simulink subsystem "AutomaticTransmissionWithTorqueConverterSSC"  (R2023b)
settings: Solver=VariableStepAuto  StartTime=0.0  StopTime=10.0  RelTol=1e-3
undefined symbols (not defined in the file): PlntTransDampVect, PlntTransEffVect, PlntTransGearNumVect, PlntTransGearRatioVect, PlntTrqConvrtrImpDamp, PlntTrqConvrtrTurbDamp
libraries: fl_lib x11, sdl_lib x5, nesl_utility x4, nesl_utility_internal x3, autolibpowerinfoutils x1, autolibsharedcommon x1
settings Model: Creator=The MathWorks, Inc.  LastModifiedBy=The MathWorks, Inc.
settings OptimizationCC: ReuseModelBlockBuffer=off
settings DebuggingCC: SubsystemReferenceDiagnosticForUnitTest=warning

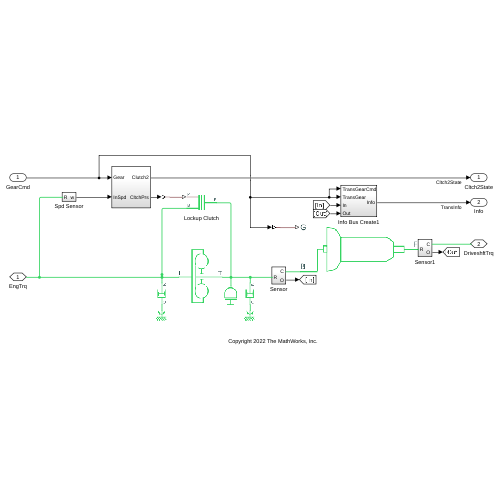
[thumbnail: Simulink's stored preview of the top-level diagram]
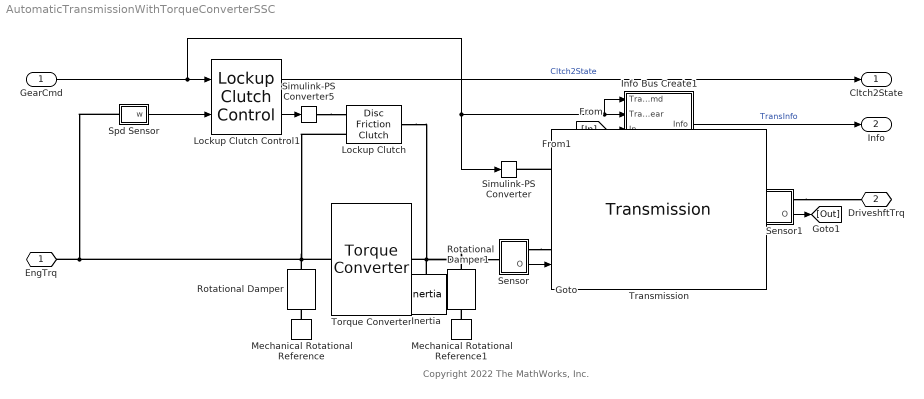
== system AutomaticTransmissionWithTorqueConverterSSC ==
  note: Copyright 2022 The MathWorks, Inc.
  GearCmd : Inport
  Inertia : fl_lib/Mechanical/Rotational Elements/Inertia  inertia=PlntTrqConvrtrTurbInertia kg*m^2  num_ports=foundation.enum.numPorts2.one  w_specify=off  w_priority=High  w=0 rad/s  w_nominal_specify=off  w_nominal_unit=rad/s  w_nominal_value=1  t_specify=off  t_priority=None  t=0 N*m  t_nominal_specify=off  t_nominal_unit=N*m  t_nominal_value=1
  Info Bus Create1 : Subsystem
  Lockup Clutch : sdl_lib/Clutches/Disc Friction Clutch  geometry_model=sdl.enum.friction_geometry.radius  r_eff=PlntTrqConvrtrCltchRadius m  d_o=150 mm  d_i=100 mm  nS=PlntTrqConvrtrCltchNumFricSurf  piston_area=PlntTrqConvrtrCltchEngdPstnArea m^2  unidirectional=sdl.enum.directionality.bidirectional  friction_model=sdl.enum.friction_model_TLU_thermal.fixed  mu_w_vector=[0, 100, 1000] rad/s  temperature_TLU=[280, 300, 320] K  mu_static=PlntTrqConvrtrCltchStatFric  mu_static_vector=[.4, .38, .36]  mu_coulomb=PlntTrqConvrtrCltchKinFric  mu_coulomb_vector=[.3, .22, .19]  mu_coulomb_temp_vector=[.3, .28, .25]  mu_coulomb_matrix=[.34, .32, .3; .3, .28, .25; .25, .2, .15]  mu_interp_method=simscape.enum.interpolation.linear  mu_extrap_method=simscape.enum.extrapolation.linear  d_f=PlntTrqConvrtrCltchDerateFctr  w_tol=PlntTrqConvrtrCltchVelTol rad/s  pressure_min=PlntTrqConvrtrCltchEngdThreshPrs Pa  mu_visc=PlntTrqConvrtrCltchViscDragTrq N*m/(rad/s)  initial_state_locked=sdl.enum.initial_lock.unlocked  enable_faults=simscape.enum.onoff.off  fault_type=sdl.enum.clutchFault.lock  external_fault=simscape.enum.onoff.off  temporal_fault=simscape.enum.onoff.off  fault_time=5 s  report_fault=simscape.enum.assert.action.none  thermal_mass=25 kJ/K  T_init=300 K
      settings: InternalSimscapePortConfiguration="{\"Bottom\":[],\"Left\":[{\"id\":\"P\",\"label\":\"P\",\"type\":\"input\"},{\"id\":\"B\",\"label\":\"B\",\"type\":\"foundation.mechanical.rotational.rotational\"}],\"Right\":[{\"id\":\"F\",\"label\":\"F\",\"type\":\"foundation.mechanical.rotational.rotational\"}],\"Top\":[]}"
  Lockup Clutch Control1 : autolibsharedcommon/Lockup Clutch Control  SystemSampleTime=-1  VariantActivationTime=update diagram  AllowFlexibleInterface=on  Latency=0  AutoFrameSizeCalculation=off
  Mechanical Rotational Reference : fl_lib/Mechanical/Rotational Elements/Mechanical Rotational Reference
  Mechanical Rotational Reference1 : fl_lib/Mechanical/Rotational Elements/Mechanical Rotational Reference
  Rotational Damper : sdl_lib/Couplings & Drives/Springs & Dampers/Rotational Damper  D=PlntTrqConvrtrImpDamp N*m*s/rad  enable_faults=simscape.enum.onoff.off  b_fault=100 N*m*s/rad  temporal_fault=simscape.enum.onoff.off  fault_time=5 s  shock_fault=simscape.enum.onoff.off  acceleration_limit=100 rad/s^2  shock_limit=1  report_fault=simscape.enum.assert.action.none  thermal_port=simscape.enum.thermaleffects.omit  thermal_mass=50 kJ/K  temperature_specify=off  temperature_priority=High  temperature=300 K  temperature_nominal_specify=off  temperature_nominal_unit=K  temperature_nominal_value=1
  Rotational Damper1 : sdl_lib/Couplings & Drives/Springs & Dampers/Rotational Damper  D=PlntTrqConvrtrTurbDamp N*m*s/rad  enable_faults=simscape.enum.onoff.off  b_fault=100 N*m*s/rad  temporal_fault=simscape.enum.onoff.off  fault_time=5 s  shock_fault=simscape.enum.onoff.off  acceleration_limit=100 rad/s^2  shock_limit=1  report_fault=simscape.enum.assert.action.none  thermal_port=simscape.enum.thermaleffects.omit  thermal_mass=50 kJ/K  temperature_specify=off  temperature_priority=High  temperature=300 K  temperature_nominal_specify=off  temperature_nominal_unit=K  temperature_nominal_value=1
  Sensor : Subsystem
      settings: PortSchema="{\"entries\":[{\"content\":{\"sides\":[{\"content\":{\"connectorIds\":[\"LConn1\"]},\"type\":\"ConnectorPlacement.EquallySpacedRectSide\",\"uuid\":\"2e27b447-89d7-4d94-b9d2-8f612a4e25ed\"},{\"content\":{\"connectorIds\":[\"RConn1\",\"Out1\"],\"side\":\"RIGHT\"},\"type\":\"ConnectorPlacement.EquallySpacedRectSide\",\"uuid\":\"d649ff29-a00c-460e-9e09-fe3bc3dd9339\"},{\"content\":{\"side\":\"TOP\"},\"type\":\"ConnectorPlacement.EquallySpacedRectSide\",\"uuid\":\"c1caa1bf-44c8-4179-bd35-f8aecae525f1\"}]},\"type\":\"ConnectorPlacement.EquallySpacedConnector\",\"uuid\":\"741ea5ec-6556-46e5-ba1b-80e523f861d6\"}],\"packageUris\":[\"http://schema.mathworks.com/mf0/Connector/R2020b\"],\"version\":\"1.0\"}"
  Sensor1 : Subsystem
      settings: PortSchema="{\"entries\":[{\"content\":{\"sides\":[{\"content\":{\"connectorIds\":[\"LConn1\"]},\"type\":\"ConnectorPlacement.EquallySpacedRectSide\",\"uuid\":\"2e27b447-89d7-4d94-b9d2-8f612a4e25ed\"},{\"content\":{\"connectorIds\":[\"RConn1\",\"Out1\"],\"side\":\"RIGHT\"},\"type\":\"ConnectorPlacement.EquallySpacedRectSide\",\"uuid\":\"d649ff29-a00c-460e-9e09-fe3bc3dd9339\"},{\"content\":{\"side\":\"TOP\"},\"type\":\"ConnectorPlacement.EquallySpacedRectSide\",\"uuid\":\"c1caa1bf-44c8-4179-bd35-f8aecae525f1\"}]},\"type\":\"ConnectorPlacement.EquallySpacedConnector\",\"uuid\":\"741ea5ec-6556-46e5-ba1b-80e523f861d6\"}],\"packageUris\":[\"http://schema.mathworks.com/mf0/Connector/R2020b\"],\"version\":\"1.0\"}"
  Simulink-PS Converter : nesl_utility_internal/Simulink-PS Converter  PhysicalDomain=network_engine_domain  SubClassName=ps_input  LeftPortType=input  RightPortType=output  PseudoPeriodic=off  Frequencies=[]  NoiseDistribution=none  NoiseParameters=[]  Unit=1  AffineConversion=off  FilteringAndDerivatives=provide  SimscapeFilterOrder=1  InputFilterTimeConstant=0.001  UdotUserProvided=0
  Simulink-PS Converter5 : nesl_utility_internal/Simulink-PS Converter  PhysicalDomain=network_engine_domain  SubClassName=ps_input  LeftPortType=input  RightPortType=output  PseudoPeriodic=off  Frequencies=[]  NoiseDistribution=none  NoiseParameters=[]  Unit=Pa  AffineConversion=off  FilteringAndDerivatives=provide  SimscapeFilterOrder=1  InputFilterTimeConstant=0.01  UdotUserProvided=0
  Spd Sensor : Subsystem
  Torque Converter : sdl_lib/Couplings & Drives/Torque Converter  coast_mode_modeling=sdl.enum.torqueConverterContinuousTwomode.continuous  SR_drive_tlu=PlntTrqConvrtrDrvModeSpdRatioVect  TR_drive_tlu=PlntTrqConvrtrDrvModeTrqRatioVect  CF_drive_tlu=PlntTrqConvrtrDrvModeCapFctrVect N*m/rpm^2  SR_coast_tlu=PlntTrqConvrtrCoastModeSpdRatioVect  CF_coast_tlu=PlntTrqConvrtrCoastModeCapFctrRatioVect N*m/rpm^2  iniMode=sdl.enum.torqueConverterInitialMode.drive  delta_w=PlntTrqConvrtrModeTransThresh rpm  n_vector=PlntTrqConvrtrSpdRatioVect  trq_vector=PlntTrqConvrtrTrqRatioVect  cf_vector_parameterization=sdl.enum.torqueConverterCFParameterization.SpeedToSqrtTorque  cf_vector_reference_speed=sdl.enum.torqueConverterCFReferenceSpeed.ImpellerSpeedAlways  cf_vector=PlntTrqConvrtrCapVect rad/(N^(1/2)*m^(1/2)*s)  cf_vector_sq=1e-3 * [6.616, 6.048, 5.787, 5.384, 4.681, 3.779, 2.671, 2.047, 1.111, .4] N*m*s^2/rad^2  interp_method=simscape.enum.interpolation.smooth  extrap_method=simscape.enum.extrapolation.nearest  model_lag=sdl.enum.torqueConverterLagOnOff.LagOff  tau=PlntTrqConvrtrTimeCnst s  initial_trq_ratio=PlntTrqConvrtrInitTrqRatio
      settings: InternalSimscapePortConfiguration="{\"Bottom\":[],\"Left\":[{\"id\":\"I\",\"label\":\"I\",\"type\":\"foundation.mechanical.rotational.rotational\"}],\"Right\":[{\"id\":\"T\",\"label\":\"T\",\"type\":\"foundation.mechanical.rotational.rotational\"}],\"Top\":[]}"
  Transmission : sdl_lib/Gears/Transmission  gear_ratios=PlntTransGearRatioVect(2:end)  reverse_ratio=PlntTransRvrseGearRatio  friction_model=sdl.enum.transmissionFriction.gear  efficiency=0.95  efficiency_tlu=PlntTransEffVect(2:end)  reverse_efficiency=PlntTransRvrseGearEff  pwr_thr=PlntTransPwrThresh W  kp=PlntTransStiff N*m/rad  kv=PlntTransDamp N*m*s/rad  initial_torque=PlntTransInitInTrq N*m  mu_visc=[PlntTransDampVect(1), PlntTransDampVect(1)] N*m*s/rad  t_friction=PlntTransCltchKinFricTrq N*m  t_locked=PlntTransCltchStatFricTrq N*m  shift_model=sdl.enum.transmissionShiftModel.instant  shift_time=PlntTransCltchShiftTime ms  w_tol=PlntTransCltchVelTol rad/s  initial_state_locked=sdl.enum.initial_lock.locked  thermal_port=simscape.enum.thermaleffects.omit  thermal_mass=100 kJ/K  initial_temperature=300 K
      settings: LogSimulationData=on  InternalSimscapePortConfiguration="{\"Bottom\":[],\"Left\":[{\"id\":\"G\",\"label\":\"G\",\"type\":\"input\"},{\"id\":\"B\",\"label\":\"B\",\"type\":\"foundation.mechanical.rotational.rotational\"}],\"Right\":[{\"id\":\"F\",\"label\":\"F\",\"type\":\"foundation.mechanical.rotational.rotational\"}],\"Top\":[]}"
  EngTrq : PMIOPort  Side=Left
  DriveshftTrq : PMIOPort  Port=2  Side=Right
  Cltch2State : Outport  VectorParamsAs1DForOutWhenUnconnected=off
  Info : Outport  Port=2  VectorParamsAs1DForOutWhenUnconnected=off
  wires:
  Info Bus Create1/1(Info) -> Info/1  "TransInfo"
  Lockup Clutch Control1/1 -> Cltch2State/1  "Cltch2State"
  GearCmd/1 -> Lockup Clutch Control1/1, Info Bus Create1/1(TransGearCmd), Info Bus Create1/2(TransGear), Simulink-PS Converter/1
  Lockup Clutch Control1/2 -> Simulink-PS Converter5/1
  Spd Sensor/1(w) -> Lockup Clutch Control1/2
  Sensor/1(O) -> [In]
  Sensor1/1(O) -> [Out]
  [In] -> Info Bus Create1/3(In)
  [Out] -> Info Bus Create1/4(Out)
  connections:
  Torque Converter/LConn1 -- Spd Sensor/LConn1 -- EngTrq/RConn1 -- Rotational Damper/LConn1 -- Lockup Clutch/LConn2
  Transmission/LConn1 -- Simulink-PS Converter/RConn1
  Mechanical Rotational Reference/LConn1 -- Rotational Damper/RConn1
  Mechanical Rotational Reference1/LConn1 -- Rotational Damper1/RConn1
  Simulink-PS Converter5/RConn1 -- Lockup Clutch/LConn1
  Lockup Clutch/RConn1 -- Rotational Damper1/LConn1 -- Sensor/LConn1 -- Torque Converter/RConn1 -- Inertia/LConn1
  Sensor1/LConn1 -- Transmission/RConn1
  Sensor/RConn1 -- Transmission/LConn2
  Sensor1/RConn1 -- DriveshftTrq/RConn1

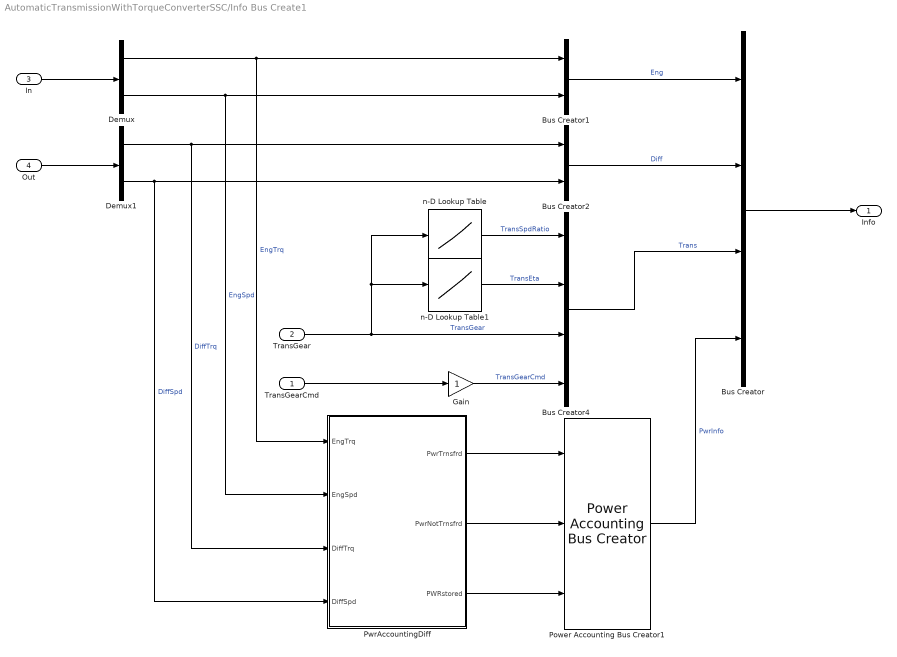
== system AutomaticTransmissionWithTorqueConverterSSC/Info Bus Create1 ==
  TransGearCmd : Inport
  TransGear : Inport  Port=2
  In : Inport  Port=3
  Out : Inport  Port=4
  Bus Creator : BusCreator  Inputs=4
  Bus Creator1 : BusCreator  Inputs=2
  Bus Creator2 : BusCreator  Inputs=2
  Bus Creator4 : BusCreator  Inputs=4
  Demux : Demux  Outputs=2
  Demux1 : Demux  Outputs=2
  Gain : Gain
  Power Accounting Bus Creator1 : autolibpowerinfoutils/Power Accounting Bus Creator  AssctBlkSelPopup=Parent  RefBlkName='libraryname/blkname'  PwrTrnsfrdCheckBox=on  PwrNotTrnsfrdCheckBox=on  PwrStoredCheckBox=on  aMode=aMode
  PwrAccountingDiff : Subsystem
  n-D Lookup Table : Lookup_n-D  NumberOfTableDimensions=1  BreakpointsForDimension1=PlntTransGearNumVect  BreakpointsForDimension3=[5, 7]  BeginIndexSearchUsingPreviousIndexResult=on  Table=PlntTransGearRatioVect  InterpMethod=Nearest  ExtrapMethod=Clip  UseLastTableValue=on  InternalRulePriority=Speed  RndMeth=Simplest
  n-D Lookup Table1 : Lookup_n-D  NumberOfTableDimensions=1  BreakpointsForDimension1=PlntTransGearNumVect  BreakpointsForDimension3=[5, 7]  BeginIndexSearchUsingPreviousIndexResult=on  Table=PlntTransEffVect  InterpMethod=Nearest  ExtrapMethod=Clip  UseLastTableValue=on  InternalRulePriority=Speed  RndMeth=Simplest
  Info : Outport
  wires:
  TransGearCmd/1 -> Gain/1
  PwrAccountingDiff/1(PwrTrnsfrd) -> Power Accounting Bus Creator1/1
  PwrAccountingDiff/3(PWRstored) -> Power Accounting Bus Creator1/3
  PwrAccountingDiff/2(PwrNotTrnsfrd) -> Power Accounting Bus Creator1/2
  Out/1 -> Demux1/1
  In/1 -> Demux/1
  Bus Creator4/1 -> Bus Creator/3  "Trans"
  Power Accounting Bus Creator1/1 -> Bus Creator/4  "PwrInfo"
  Demux1/2 -> Bus Creator2/2, PwrAccountingDiff/4(DiffSpd)  "DiffSpd"
  n-D Lookup Table1/1 -> Bus Creator4/2  "TransEta"
  Bus Creator1/1 -> Bus Creator/1  "Eng"
  Demux/2 -> Bus Creator1/2, PwrAccountingDiff/2(EngSpd)  "EngSpd"
  Demux1/1 -> Bus Creator2/1, PwrAccountingDiff/3(DiffTrq)  "DiffTrq"
  Bus Creator/1 -> Info/1
  n-D Lookup Table/1 -> Bus Creator4/1  "TransSpdRatio"
  Demux/1 -> Bus Creator1/1, PwrAccountingDiff/1(EngTrq)  "EngTrq"
  TransGear/1 -> n-D Lookup Table/1, n-D Lookup Table1/1, Bus Creator4/3  "TransGear"
  Bus Creator2/1 -> Bus Creator/2  "Diff"
  Gain/1 -> Bus Creator4/4  "TransGearCmd"

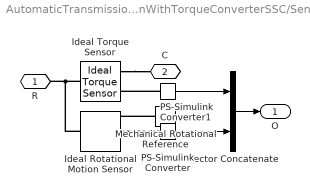
== system AutomaticTransmissionWithTorqueConverterSSC/Sensor ==
  Ideal Rotational Motion Sensor : fl_lib/Mechanical/Mechanical Sensors/Ideal Rotational Motion Sensor  reference=foundation.enum.MeasurementReference.difference  acceleration_port=false  velocity_port=true  position_port=true  wrap_angle=false  offset=0 rad
  Ideal Torque Sensor : fl_lib/Mechanical/Mechanical Sensors/Ideal Torque Sensor
  Mechanical Rotational Reference : fl_lib/Mechanical/Rotational Elements/Mechanical Rotational Reference
  PS-Simulink Converter : nesl_utility/PS-Simulink Converter  PhysicalDomain=network_engine_domain  SubClassName=ps_output  LeftPortType=input  RightPortType=output  PseudoPeriodic=off  Frequencies=[]  VectorFormat=inherit  Unit=inherit  AffineConversion=off
  PS-Simulink Converter1 : nesl_utility/PS-Simulink Converter  PhysicalDomain=network_engine_domain  SubClassName=ps_output  LeftPortType=input  RightPortType=output  PseudoPeriodic=off  Frequencies=[]  VectorFormat=inherit  Unit=inherit  AffineConversion=off
  Vector Concatenate : Concatenate
  R : PMIOPort  Side=Left
  C : PMIOPort  Port=2  Side=Right
  O : Outport
  wires:
  PS-Simulink Converter1/1 -> Vector Concatenate/1
  PS-Simulink Converter/1 -> Vector Concatenate/2
  Vector Concatenate/1 -> O/1
  connections:
  PS-Simulink Converter1/LConn1 -- Ideal Torque Sensor/RConn2
  Ideal Torque Sensor/LConn1 -- Ideal Rotational Motion Sensor/LConn1 -- R/RConn1
  Ideal Torque Sensor/RConn1 -- C/RConn1
  Mechanical Rotational Reference/LConn1 -- Ideal Rotational Motion Sensor/RConn1
  PS-Simulink Converter/LConn1 -- Ideal Rotational Motion Sensor/RConn2

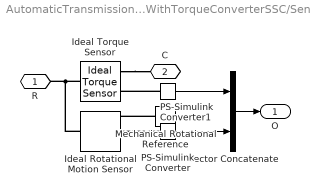
== system AutomaticTransmissionWithTorqueConverterSSC/Sensor1 ==
  Ideal Rotational Motion Sensor : fl_lib/Mechanical/Mechanical Sensors/Ideal Rotational Motion Sensor  reference=foundation.enum.MeasurementReference.difference  acceleration_port=false  velocity_port=true  position_port=true  wrap_angle=false  offset=0 rad
  Ideal Torque Sensor : fl_lib/Mechanical/Mechanical Sensors/Ideal Torque Sensor
  Mechanical Rotational Reference : fl_lib/Mechanical/Rotational Elements/Mechanical Rotational Reference
  PS-Simulink Converter : nesl_utility/PS-Simulink Converter  PhysicalDomain=network_engine_domain  SubClassName=ps_output  LeftPortType=input  RightPortType=output  PseudoPeriodic=off  Frequencies=[]  VectorFormat=inherit  Unit=inherit  AffineConversion=off
  PS-Simulink Converter1 : nesl_utility/PS-Simulink Converter  PhysicalDomain=network_engine_domain  SubClassName=ps_output  LeftPortType=input  RightPortType=output  PseudoPeriodic=off  Frequencies=[]  VectorFormat=inherit  Unit=inherit  AffineConversion=off
  Vector Concatenate : Concatenate
  R : PMIOPort  Side=Left
  C : PMIOPort  Port=2  Side=Right
  O : Outport
  wires:
  Vector Concatenate/1 -> O/1
  PS-Simulink Converter/1 -> Vector Concatenate/2
  PS-Simulink Converter1/1 -> Vector Concatenate/1
  connections:
  PS-Simulink Converter/LConn1 -- Ideal Rotational Motion Sensor/RConn2
  Mechanical Rotational Reference/LConn1 -- Ideal Rotational Motion Sensor/RConn1
  Ideal Torque Sensor/RConn1 -- C/RConn1
  Ideal Rotational Motion Sensor/LConn1 -- Ideal Torque Sensor/LConn1 -- R/RConn1
  PS-Simulink Converter1/LConn1 -- Ideal Torque Sensor/RConn2

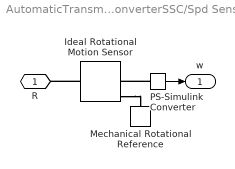
== system AutomaticTransmissionWithTorqueConverterSSC/Spd Sensor ==
  Ideal Rotational Motion Sensor : fl_lib/Mechanical/Mechanical Sensors/Ideal Rotational Motion Sensor  reference=foundation.enum.MeasurementReference.difference  acceleration_port=false  velocity_port=true  position_port=true  wrap_angle=simscape.enum.onoff.off  offset=0 rad
  Mechanical Rotational Reference : fl_lib/Mechanical/Rotational Elements/Mechanical Rotational Reference
  PS-Simulink Converter : nesl_utility_internal/PS-Simulink Converter  PhysicalDomain=network_engine_domain  SubClassName=ps_output  LeftPortType=input  RightPortType=output  PseudoPeriodic=off  Frequencies=[]  VectorFormat=inherit  Unit=inherit  AffineConversion=off
  R : PMIOPort  Side=Left
  w : Outport
  wires:
  PS-Simulink Converter/1 -> w/1
  connections:
  PS-Simulink Converter/LConn1 -- Ideal Rotational Motion Sensor/RConn2
  Ideal Rotational Motion Sensor/LConn1 -- R/RConn1
  Ideal Rotational Motion Sensor/RConn1 -- Mechanical Rotational Reference/LConn1

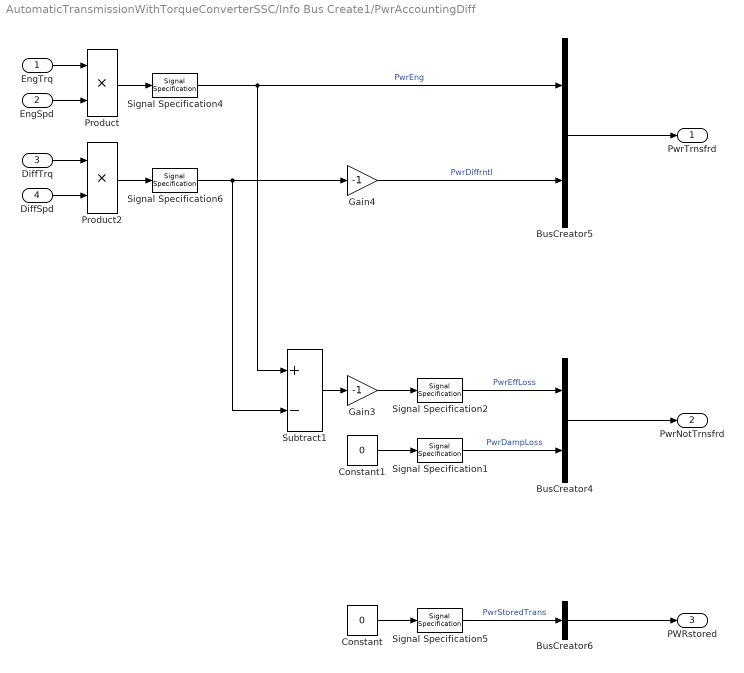
== system AutomaticTransmissionWithTorqueConverterSSC/Info Bus Create1/PwrAccountingDiff ==
  EngTrq : Inport
  EngSpd : Inport  Port=2
  DiffTrq : Inport  Port=3
  DiffSpd : Inport  Port=4
  BusCreator4 : BusCreator  Inputs=2
  BusCreator5 : BusCreator  Inputs=2
  BusCreator6 : BusCreator  Inputs=1
  Constant : Constant  Value=0  SampleTime=-1
  Constant1 : Constant  Value=0  SampleTime=-1
  Gain3 : Gain  Gain=-1
  Gain4 : Gain  Gain=-1
  Product : Product
  Product2 : Product
  Signal Specification{1..2,4..6} (5 alike) : SignalSpecification  Unit=W
  Subtract1 : Sum  Inputs=+-
  PwrTrnsfrd : Outport
  PwrNotTrnsfrd : Outport  Port=2
  PWRstored : Outport  Port=3
  wires:
  Signal Specification1/1 -> BusCreator4/2  "PwrDampLoss"
  Constant1/1 -> Signal Specification1/1
  BusCreator5/1 -> PwrTrnsfrd/1
  BusCreator6/1 -> PWRstored/1
  DiffTrq/1 -> Product2/1
  EngSpd/1 -> Product/2
  BusCreator4/1 -> PwrNotTrnsfrd/1
  Subtract1/1 -> Gain3/1
  Signal Specification6/1 -> Gain4/1, Subtract1/2
  Signal Specification5/1 -> BusCreator6/1  "PwrStoredTrans"
  Gain4/1 -> BusCreator5/2  "PwrDiffrntl"
  Signal Specification4/1 -> Subtract1/1, BusCreator5/1  "PwrEng"
  Gain3/1 -> Signal Specification2/1
  DiffSpd/1 -> Product2/2
  Signal Specification2/1 -> BusCreator4/1  "PwrEffLoss"
  Product2/1 -> Signal Specification6/1
  EngTrq/1 -> Product/1
  Product/1 -> Signal Specification4/1
  Constant/1 -> Signal Specification5/1
